simulink model "control"  (R2022b)
settings: Solver=VariableStepAuto  StartTime=0.0  StopTime=4.0  FixedStep=0.001  MaxStep=0.1  RelTol=1e-3
values from neighbouring files (symbols this model uses):
  q_values = [-0.927293431584587;-1.28700579042062;0.700000000000000;2.21429922200521]    [init.m]
undefined symbols (not defined in the file or in its folder): DiscIntNeverNeededParam, Ts
settings Model: Creator=giuseppeloianno  LastModifiedBy=DELL

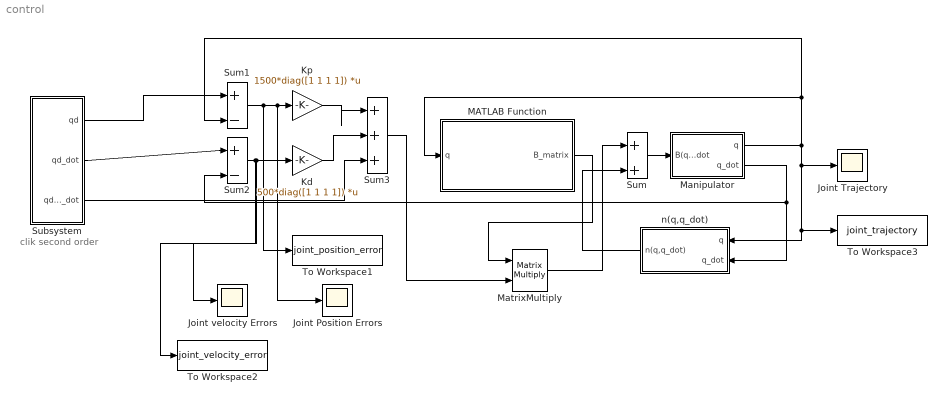
== system control ==
  note: clik second order
  Joint Position Errors : Scope
  Joint Trajectory : Scope
  Joint velocity Errors : Scope
  Kd : Gain  Gain=500*diag([1 1 1 1])  Multiplication=Matrix(K*u)
  Kp : Gain  Gain=1500*diag([1 1 1 1])  Multiplication=Matrix(K*u)
  MATLAB Function : MATLAB Function  TreatAsAtomicUnit=on
  Manipulator : Subsystem
  MatrixMultiply : Product  Multiplication=Matrix(*)
  Subsystem : Subsystem
  Sum : Sum  Inputs=|++
  Sum1 : Sum  Inputs=|+-
  Sum2 : Sum  Inputs=|+-
  Sum3 : Sum  Inputs=|+++
  To Workspace1 : ToWorkspace  VariableName=joint_position_error  SampleTime=Ts
  To Workspace2 : ToWorkspace  VariableName=joint_velocity_error  SampleTime=Ts
  To Workspace3 : ToWorkspace  VariableName=joint_trajectory  SampleTime=Ts
  n(q,q_dot) : Subsystem
  wires:
  n(q,q_dot)/1(n(q,q_dot)) -> Sum/2
  Kd/1 -> Sum3/2
  Sum2/1 -> Kd/1, Joint velocity Errors/1, To Workspace2/1
  Sum1/1 -> To Workspace1/1, Joint Position Errors/1, Kp/1
  Kp/1 -> Sum3/1
  Manipulator/1(q) -> Joint Trajectory/1, To Workspace3/1, n(q,q_dot)/1(q), Sum1/2, MATLAB Function/1(q)
  Manipulator/2(q_dot) -> Sum2/2, n(q,q_dot)/2(q_dot)
  Subsystem/1(qd) -> Sum1/1
  Subsystem/2(qd_dot) -> Sum2/1
  Sum3/1 -> MatrixMultiply/2
  Sum/1 -> Manipulator/1(B(q)q_dot_dot)
  Subsystem/3(qd_dot_dot) -> Sum3/3
  MATLAB Function/1(B_matrix) -> MatrixMultiply/1
  MatrixMultiply/1 -> Sum/1

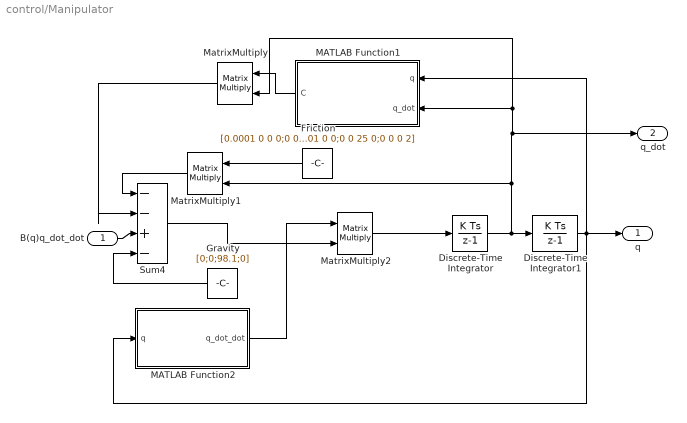
== system control/Manipulator ==
  B(q)q_dot_dot : Inport
  Discrete-Time Integrator : DiscreteIntegrator  SampleTime=Ts  ICPrevOutput=DiscIntNeverNeededParam  ICPrevScaledInput=DiscIntNeverNeededParam
  Discrete-Time Integrator1 : DiscreteIntegrator  InitialCondition=q_values  SampleTime=Ts  LimitOutput=on  UpperSaturationLimit=[pi/2;pi/4;1;2*pi]  LowerSaturationLimit=[-pi/2;-pi/2;0.25;-2*pi]  ICPrevOutput=DiscIntNeverNeededParam  ICPrevScaledInput=DiscIntNeverNeededParam
  Friction : Constant  Value=[0.0001 0 0 0;0 0.0001 0 0;0 0 25 0;0 0 0 2]
  Gravity : Constant  Value=[0;0;98.1;0]
  MATLAB Function1 : MATLAB Function  TreatAsAtomicUnit=on
  MATLAB Function2 : MATLAB Function  TreatAsAtomicUnit=on
  MatrixMultiply : Product  Multiplication=Matrix(*)
  MatrixMultiply1 : Product  Multiplication=Matrix(*)
  MatrixMultiply2 : Product  Multiplication=Matrix(*)
  Sum4 : Sum  Inputs=|--+-
  q : Outport
  q_dot : Outport  Port=2
  wires:
  Discrete-Time Integrator/1 -> Discrete-Time Integrator1/1, q_dot/1, MatrixMultiply/2, MATLAB Function1/2(q_dot), MatrixMultiply1/2
  B(q)q_dot_dot/1 -> Sum4/3
  Discrete-Time Integrator1/1 -> q/1, MATLAB Function1/1(q), MATLAB Function2/1(q)
  MatrixMultiply/1 -> Sum4/2
  Friction/1 -> MatrixMultiply1/1
  MatrixMultiply1/1 -> Sum4/1
  MatrixMultiply2/1 -> Discrete-Time Integrator/1
  Gravity/1 -> Sum4/4
  MATLAB Function1/1(C) -> MatrixMultiply/1
  MATLAB Function2/1(q_dot_dot) -> MatrixMultiply2/1
  Sum4/1 -> MatrixMultiply2/2

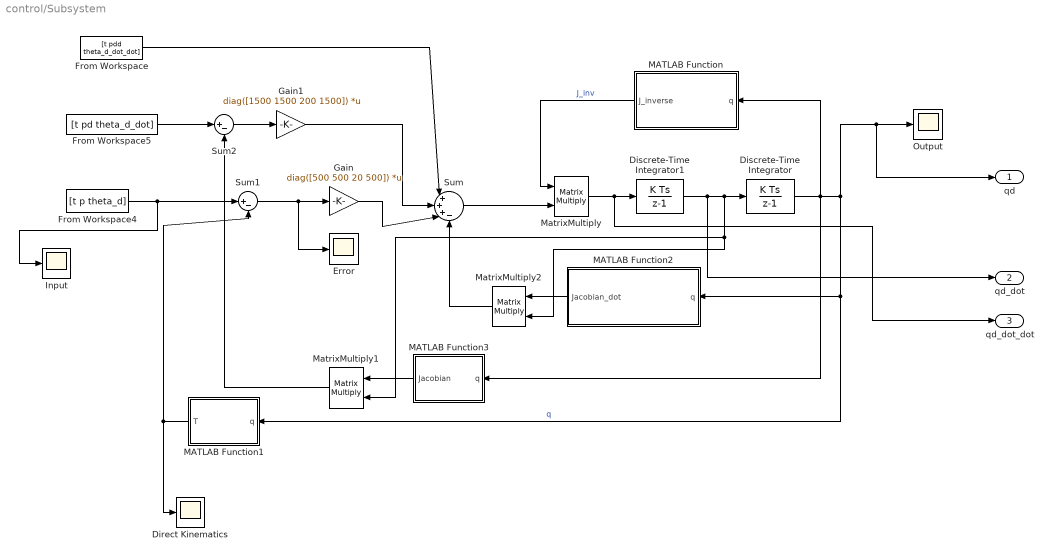
== system control/Subsystem ==
  Direct Kinematics : Scope
  Discrete-Time Integrator : DiscreteIntegrator  InitialCondition=q_values  SampleTime=Ts  LimitOutput=on  UpperSaturationLimit=[pi/2;pi/4;1;2*pi]  LowerSaturationLimit=[-pi/2;-pi/2;0.25;-2*pi]  ICPrevOutput=DiscIntNeverNeededParam  ICPrevScaledInput=DiscIntNeverNeededParam
  Discrete-Time Integrator1 : DiscreteIntegrator  SampleTime=Ts  UpperSaturationLimit=[pi/2;pi/4;1;2*pi]  LowerSaturationLimit=[-pi/2;-pi/2;0.25;-2*pi]  ICPrevOutput=DiscIntNeverNeededParam  ICPrevScaledInput=DiscIntNeverNeededParam
  Error : Scope
  From Workspace : FromWorkspace  VariableName=[t pdd theta_d_dot_dot]  SampleTime=Ts
  From Workspace4 : FromWorkspace  VariableName=[t p theta_d]  SampleTime=Ts
  From Workspace5 : FromWorkspace  VariableName=[t pd theta_d_dot]  SampleTime=Ts
  Gain : Gain  Gain=diag([500 500 20 500])  Multiplication=Matrix(K*u)
  Gain1 : Gain  Gain=diag([1500 1500 200 1500])  Multiplication=Matrix(K*u)
  Input : Scope
  MATLAB Function : MATLAB Function  TreatAsAtomicUnit=on
  MATLAB Function1 : MATLAB Function  TreatAsAtomicUnit=on
  MATLAB Function2 : MATLAB Function  TreatAsAtomicUnit=on
  MATLAB Function3 : MATLAB Function  TreatAsAtomicUnit=on
  MatrixMultiply : Product  Multiplication=Matrix(*)
  MatrixMultiply1 : Product  Multiplication=Matrix(*)
  MatrixMultiply2 : Product  Multiplication=Matrix(*)
  Output : Scope
  Sum : Sum  Inputs=|+++-
  Sum1 : Sum  Inputs=|+-
  Sum2 : Sum  Inputs=|+-
  qd : Outport
  qd_dot : Outport  Port=2
  qd_dot_dot : Outport  Port=3
  wires:
  Gain/1 -> Sum/3
  Sum2/1 -> Gain1/1
  Discrete-Time Integrator/1 -> MATLAB Function/1(q), MATLAB Function3/1(q), MATLAB Function2/1(q), MATLAB Function1/1(q), qd/1, Output/1  "q"
  MATLAB Function3/1(Jacobian) -> MatrixMultiply1/1
  Gain1/1 -> Sum/2
  From Workspace/1 -> Sum/1
  MATLAB Function2/1(Jacobian_dot) -> MatrixMultiply2/1
  Sum1/1 -> Error/1, Gain/1
  Sum/1 -> MatrixMultiply/2
  MatrixMultiply2/1 -> Sum/4
  From Workspace4/1 -> Input/1, Sum1/1
  MATLAB Function1/1(T) -> Direct Kinematics/1, Sum1/2
  Discrete-Time Integrator1/1 -> qd_dot/1, MatrixMultiply2/2, MatrixMultiply1/2, Discrete-Time Integrator/1
  From Workspace5/1 -> Sum2/1
  MatrixMultiply1/1 -> Sum2/2
  MATLAB Function/1(J_inverse) -> MatrixMultiply/1  "J_inv"
  MatrixMultiply/1 -> qd_dot_dot/1, Discrete-Time Integrator1/1

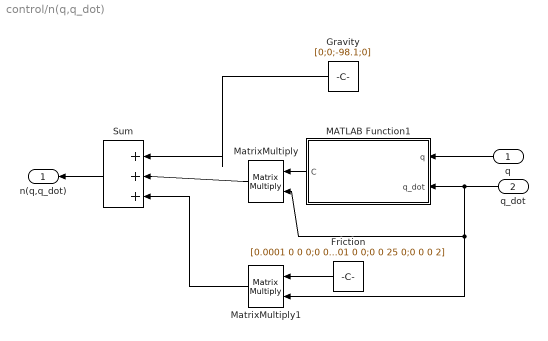
== system control/n(q,q_dot) ==
  q : Inport
  q_dot : Inport  Port=2
  Friction : Constant  Value=[0.0001 0 0 0;0 0.0001 0 0;0 0 25 0;0 0 0 2]
  Gravity : Constant  Value=[0;0;-98.1;0]
  MATLAB Function1 : MATLAB Function  TreatAsAtomicUnit=on
  MatrixMultiply : Product  Multiplication=Matrix(*)
  MatrixMultiply1 : Product  Multiplication=Matrix(*)
  Sum : Sum  Inputs=|+++
  n(q,q_dot) : Outport
  wires:
  q/1 -> MATLAB Function1/1(q)
  Sum/1 -> n(q,q_dot)/1
  Gravity/1 -> Sum/1
  MATLAB Function1/1(C) -> MatrixMultiply/1
  q_dot/1 -> MatrixMultiply1/2, MatrixMultiply/2, MATLAB Function1/2(q_dot)
  MatrixMultiply/1 -> Sum/2
  MatrixMultiply1/1 -> Sum/3
  Friction/1 -> MatrixMultiply1/1

== matlab function control/n(q,q_dot)/MATLAB Function1 ==
  data: q input; q_dot input; C output
function C = C_matrix(q, q_dot)

%Defining the required parameters
a1 = 05;
a2 = 0.5;
l2 = 0.25;
m_l2 = 25;
m_l3 = 15;

%Initialzing the C matrix
C = zeros(4,4);

%Assigning values to each row and column of the C matrix
C(1,1) = (-m_l2*a1*l2*sin(q(2)) - m_l3*a1*a2*sin(q(2))).*q_dot(2);

C(1,2) = (-m_l2*a1*l2*sin(q(2)) - m_l3*a1*a2*sin(q(2))).*(q_dot(1)+q_dot(2));

C(2,1) = -((-m_l2*a1*l2*sin(q(2)) - m_l3*a1*a2*sin(q(2))).*q_dot(1));

end

== matlab function control/MATLAB Function ==
  data: q input; B_matrix output
function B_matrix = inertia(q)

%Calling the B function which generates the Inertia matrix 
B_matrix = B(q); 

end

== matlab function control/Subsystem/MATLAB Function ==
  data: q input; J_inverse output
function J_inverse = jacobian_inverse(q)

% Calling the jacobian function from the jacobian matlab file
J = jacobian(q);

% Calculating inverse of jacobian matrix
J_inverse = inv(J);

== matlab function control/Manipulator/MATLAB Function1 ==
  data: q input; q_dot input; C output
function C = C_matrix(q, q_dot)

%Defining the required parameters
a1 = 0.5;
a2 = 0.5;
l2 = 0.25;
m_l2 = 25;
m_l3 = 15;

%Initialzing the C matrix
C = zeros(4,4);

%Assigning values to each row and column of the C matrix
C(1,1) = (-m_l2*a1*l2*sin(q(2)) - m_l3*a1*a2*sin(q(2))).*q_dot(2);

C(1,2) = (-m_l2*a1*l2*sin(q(2)) - m_l3*a1*a2*sin(q(2))).*(q_dot(1)+q_dot(2));

C(2,1) = -((-m_l2*a1*l2*sin(q(2)) - m_l3*a1*a2*sin(q(2))).*q_dot(1));

end

== matlab function control/Manipulator/MATLAB Function2 ==
  data: q input; q_dot_dot output
function q_dot_dot = Bq_inverse(q)

%Calling the B function which generates the Inertia matrix 
B_matrix = B(q); 

%Taking inverse of the B_matrix
q_dot_dot = inv(B_matrix);

end

== matlab function control/Subsystem/MATLAB Function1 ==
  data: q input; T output
function T = direct_kin(q)

% Defining link length values
a1 = 0.5;
a2 = 0.5;
d0 = 1;

% Assigning individual joint values to the corresponding rows of the
% q(angle) being taken as input
q1=q(1);
q2=q(2);
d3=q(3);
q4=q(4);

% Obtained Rotation and translation direct kinematics matrix for scara manipulator
R=[cos(q1+q2+q4),sin(q1+q2+q4),0;sin(q1+q2+q4),-cos(q1+q2+q4),0;0,0,-1;0 0 0];
T=[a1*cos(q1)+a2*cos(q1+q2);a1*sin(q1)+a2*sin(q1+q2);-d3+d0;0];

== matlab function control/Subsystem/MATLAB Function2 ==
  data: q input; Jacobian_dot output
function Jacobian_dot = jacobian_dot(q)

% Calling the jacobian_dot function which finds first order differential of
% jacobian matrix
Jacobian_dot = jacobian_dot(q);

== matlab function control/Subsystem/MATLAB Function3 ==
  data: q input; Jacobian output
function Jacobian = jacobian(q)

% Calling the jacobian function to get the jacobian matrix
Jacobian = jacobian(q);
